simulink model "Electronic_Throttle_Control_Failure_Model"  (R2024a)
settings: Solver=FixedStepAuto  StartTime=0.0  StopTime=2  RelTol=1e-3
libraries: simulink x5, SignalEditorBlockLib x1
settings Model: Creator=DELL  LastModifiedBy=DELL

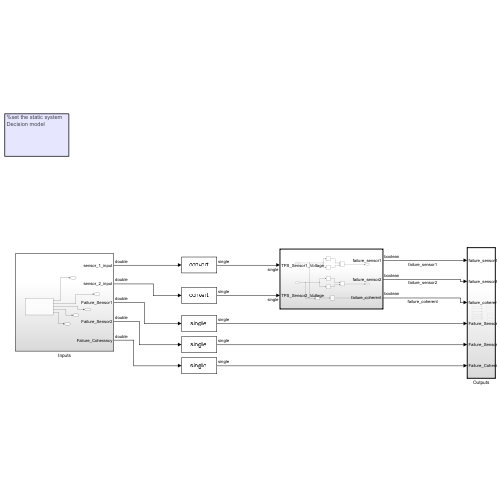
[thumbnail: Simulink's stored preview of the top-level diagram]
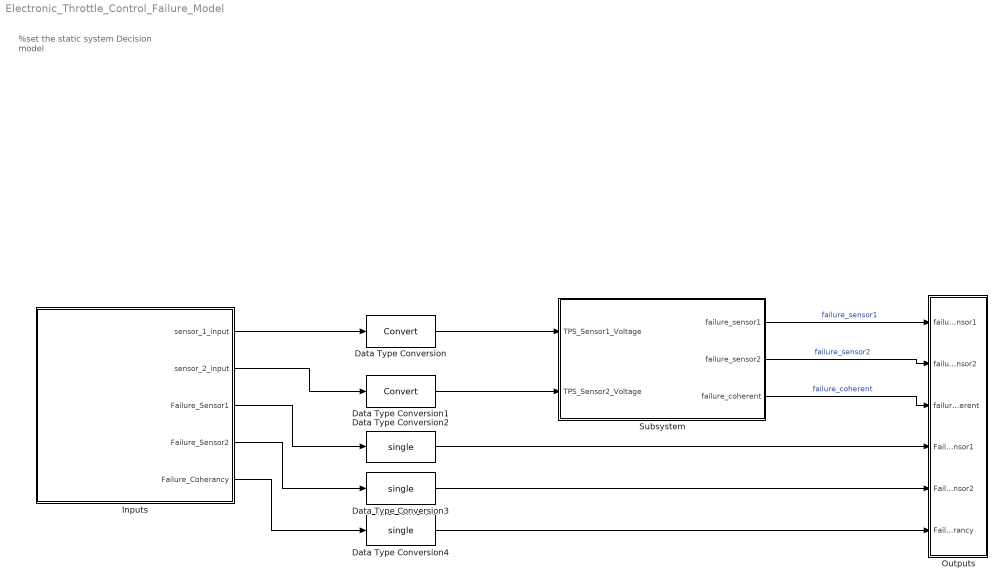
== system Electronic_Throttle_Control_Failure_Model ==
  note: %set the static system
      | Decision model
  Data Type Conversion : DataTypeConversion  SaturateOnIntegerOverflow=off  RndMeth=Floor
  Data Type Conversion1 : DataTypeConversion  SaturateOnIntegerOverflow=off  RndMeth=Floor
  Data Type Conversion2 : DataTypeConversion  OutDataTypeStr=single  SaturateOnIntegerOverflow=off  RndMeth=Floor
  Data Type Conversion3 : DataTypeConversion  OutDataTypeStr=single  SaturateOnIntegerOverflow=off  RndMeth=Floor
  Data Type Conversion4 : DataTypeConversion  OutDataTypeStr=single  SaturateOnIntegerOverflow=off  RndMeth=Floor
  Inputs : Subsystem
  Outputs : Subsystem  TreatAsAtomicUnit=on
  Subsystem : Subsystem  TreatAsAtomicUnit=on
  wires:
  Data Type Conversion/1 -> Subsystem/1(TPS_Sensor1_Voltage)
  Data Type Conversion1/1 -> Subsystem/2(TPS_Sensor2_Voltage)
  Subsystem/1(failure_sensor1) -> Outputs/1(failure_sensor1)  "failure_sensor1"
  Subsystem/2(failure_sensor2) -> Outputs/2(failure_sensor2)  "failure_sensor2"
  Subsystem/3(failure_coherent) -> Outputs/3(failure_coherent)  "failure_coherent"
  Inputs/1(sensor_1_input) -> Data Type Conversion/1
  Inputs/2(sensor_2_input) -> Data Type Conversion1/1
  Inputs/3(Failure_Sensor1) -> Data Type Conversion2/1
  Inputs/4(Failure_Sensor2) -> Data Type Conversion3/1
  Inputs/5(Failure_Coherancy) -> Data Type Conversion4/1
  Data Type Conversion2/1 -> Outputs/4(Failure_Sensor1)
  Data Type Conversion3/1 -> Outputs/5(Failure_Sensor2)
  Data Type Conversion4/1 -> Outputs/6(Failure_Coherancy)

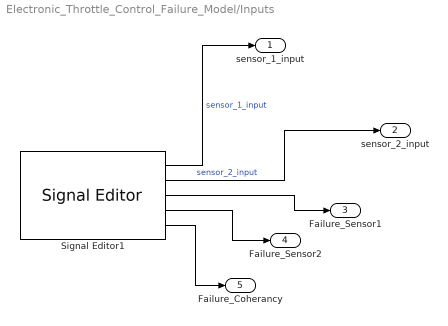
== system Electronic_Throttle_Control_Failure_Model/Inputs ==
  Signal Editor1 : SignalEditorBlockLib/Signal Editor  FileName=Test_TPS.mat  ActiveScenario=Sheet2  ActiveSignal=TPS_Sensor1_Voltage  IsBus=off  OutputBusObjectStr=Bus: BusObject  SampleTime=0  Interpolate=off  ZeroCross=off  OutputAfterFinalValue=Setting to zero  Unit=inherit  PreserveSignalName=on  ApplySigPropsToAllScenarios=on  ApplySigPropsToAllSignals=off
  sensor_1_input : Outport
  sensor_2_input : Outport  Port=2
  Failure_Sensor1 : Outport  Port=3
  Failure_Sensor2 : Outport  Port=4
  Failure_Coherancy : Outport  Port=5
  wires:
  Signal Editor1/2 -> sensor_2_input/1  "sensor_2_input"
  Signal Editor1/1 -> sensor_1_input/1  "sensor_1_input"
  Signal Editor1/5 -> Failure_Coherancy/1
  Signal Editor1/3 -> Failure_Sensor1/1
  Signal Editor1/4 -> Failure_Sensor2/1

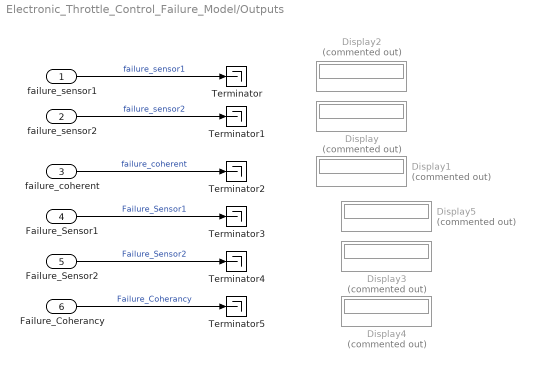
== system Electronic_Throttle_Control_Failure_Model/Outputs ==
  failure_sensor1 : Inport
  failure_sensor2 : Inport  Port=2
  failure_coherent : Inport  Port=3
  Failure_Sensor1 : Inport  Port=4
  Failure_Sensor2 : Inport  Port=5
  Failure_Coherancy : Inport  Port=6
  Display{,1..5} (6 alike) : Display  Commented=on
  Terminator{,1..5} (6 alike) : Terminator
  wires:
  failure_sensor2/1 -> Terminator1/1  "failure_sensor2"
  failure_sensor1/1 -> Terminator/1  "failure_sensor1"
  failure_coherent/1 -> Terminator2/1  "failure_coherent"
  Failure_Sensor1/1 -> Terminator3/1  "Failure_Sensor1"
  Failure_Coherancy/1 -> Terminator5/1  "Failure_Coherancy"
  Failure_Sensor2/1 -> Terminator4/1  "Failure_Sensor2"

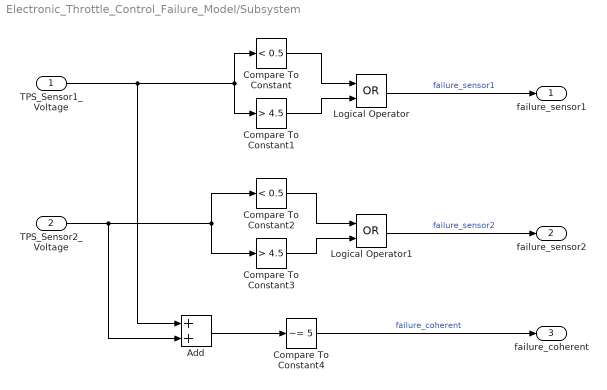
== system Electronic_Throttle_Control_Failure_Model/Subsystem ==
  TPS_Sensor1_Voltage : Inport  OutDataTypeStr=single
  TPS_Sensor2_Voltage : Inport  Port=2  OutDataTypeStr=single
  Add : Sum
  Compare To Constant : simulink/Logic and Bit Operations/Compare To Constant  relop=<  const=0.5  OutDataTypeStr=boolean
  Compare To Constant1 : simulink/Logic and Bit Operations/Compare To Constant  relop=>  const=4.5  OutDataTypeStr=boolean
  Compare To Constant2 : simulink/Logic and Bit Operations/Compare To Constant  relop=<  const=0.5  OutDataTypeStr=boolean
  Compare To Constant3 : simulink/Logic and Bit Operations/Compare To Constant  relop=>  const=4.5  OutDataTypeStr=boolean  ZeroCross=off
  Compare To Constant4 : simulink/Logic and Bit Operations/Compare To Constant  relop=~=  const=5  OutDataTypeStr=boolean
  Logical Operator : Logic  Operator=OR  AllPortsSameDT=off  OutDataTypeStr=boolean
  Logical Operator1 : Logic  Operator=OR  AllPortsSameDT=off  OutDataTypeStr=boolean
  failure_sensor1 : Outport  OutDataTypeStr=boolean
  failure_sensor2 : Outport  Port=2  OutDataTypeStr=boolean
  failure_coherent : Outport  Port=3  OutDataTypeStr=boolean
  wires:
  Compare To Constant/1 -> Logical Operator/1
  Compare To Constant1/1 -> Logical Operator/2
  Logical Operator/1 -> failure_sensor1/1  "failure_sensor1"
  TPS_Sensor1_Voltage/1 -> Add/1, Compare To Constant/1, Compare To Constant1/1
  TPS_Sensor2_Voltage/1 -> Add/2, Compare To Constant3/1, Compare To Constant2/1
  Compare To Constant2/1 -> Logical Operator1/1
  Compare To Constant3/1 -> Logical Operator1/2
  Logical Operator1/1 -> failure_sensor2/1  "failure_sensor2"
  Add/1 -> Compare To Constant4/1
  Compare To Constant4/1 -> failure_coherent/1  "failure_coherent"
